simulink model "simultaneous_amp_freq_modulation_simulink"  (R2019a)
settings: Solver=VariableStepAuto  StartTime=0.0  StopTime=10.0  RelTol=1e-3
values from neighbouring files (symbols this model uses):
  fs = 1/Ts    (= 2560)    [Simultaneous_Amp_and_Freq_Modulation_2.m]    (also in Time_Frequency_Power_domain_analysis.m = 850; extended_spectral_analysis.m)
  m = 0.25    [Simultaneous_Amp_and_Freq_Modulation_2.m]    (also in Time_Frequency_Power_domain_analysis.m = 0.5; extended_spectral_analysis.m)
libraries: dspxfrm3 x2, dspsrcs4 x1
settings Model: Creator=HP  LastModifiedBy=PRASHANT
settings DataIOCC: ReturnWorkspaceOutputs=off
settings DebuggingCC: PregeneratedLibrarySubsystemCodeDiagnostic=none  ArithmeticOperatorsInVariantConditions=warning
settings SFSimCC: SimUseLocalCustomCode=off
settings RTWCC: RTWUseLocalCustomCode=off

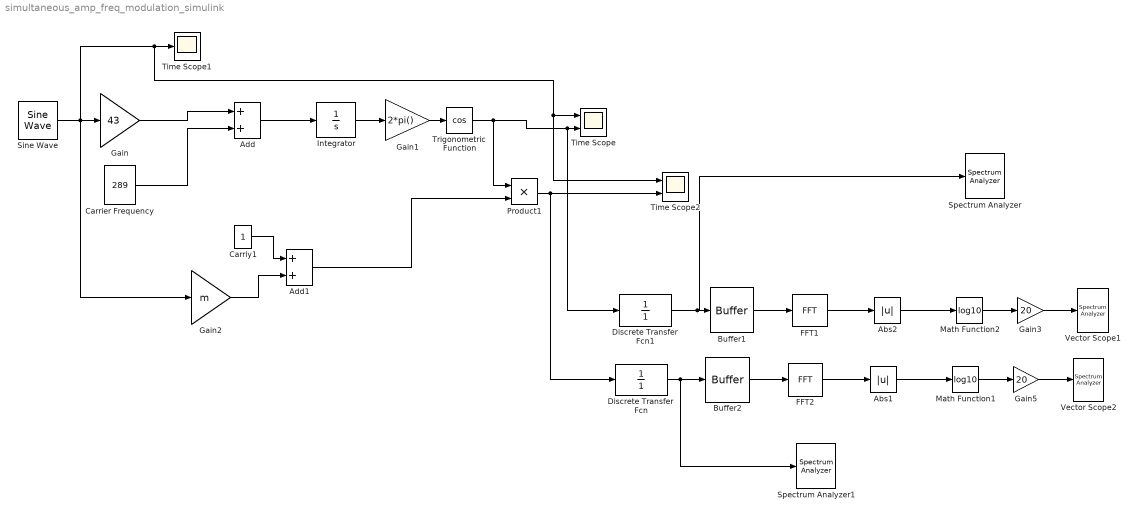
== system simultaneous_amp_freq_modulation_simulink ==
  Abs1 : Abs
  Abs2 : Abs
  Add : Sum
  Add1 : Sum
  Buffer1 : Buffer  N=4096*4
  Buffer2 : Buffer  N=4096*4
  Carrier Frequency : Constant  Value=289
  Carriy1 : Constant
  Discrete Transfer Fcn : DiscreteTransferFcn  Denominator=[1]  SampleTime=1/fs
  Discrete Transfer Fcn1 : DiscreteTransferFcn  Denominator=[1]  SampleTime=1/fs
  FFT1 : dspxfrm3/FFT  FFTImplementation=Auto  CompMethod=Table lookup  TableOpt=NEW  TableOptActive=Speed  BitRevOrder=off  Normalize=on  InheritFFTLength=off  FFTLength=4096  WrapInput=on  roundingMode=Floor  overflowMode=off  firstCoeffDataTypeStr=Inherit: Same word length as input  firstCoeffLastDataTypeStr=Inherit: Same word length as input  outputMin=[]  outputMax=[]
  FFT2 : dspxfrm3/FFT  FFTImplementation=Auto  CompMethod=Table lookup  TableOpt=NEW  TableOptActive=Speed  BitRevOrder=off  Normalize=on  InheritFFTLength=off  FFTLength=4096  WrapInput=on  roundingMode=Floor  overflowMode=off  firstCoeffDataTypeStr=Inherit: Same word length as input  firstCoeffLastDataTypeStr=Inherit: Same word length as input  outputMin=[]  outputMax=[]
  Gain : Gain  Gain=43
  Gain1 : Gain  Gain=2*pi()
  Gain2 : Gain  Gain=m
  Gain3 : Gain  Gain=20
  Gain5 : Gain  Gain=20
  Integrator : Integrator
  Math Function1 : Math  Operator=log10  SaturateOnIntegerOverflow=on
  Math Function2 : Math  Operator=log10  SaturateOnIntegerOverflow=on
  Product1 : Product
  Sine Wave : dspsrcs4/Sine Wave  Amplitude=2  Frequency=50  Phase=0  SampleMode=Discrete  OutComplex=Real  CompMethod=Trigonometric fcn  TableSize=Speed  SampleTime=1/fs  SamplesPerFrame=1  ResetState=Restart at time zero  OutputFrames=off  dataType=double  wordLen=16  udDataType=sfix(16)  fracBitsMode=Best precision  numFracBits=15  OutDataTypeStr=double  LastOutDataTypeStr=double
  Spectrum Analyzer : SpectrumAnalyzer
  Spectrum Analyzer1 : SpectrumAnalyzer
  Time Scope : Scope  NumInputPorts=2
  Time Scope1 : Scope
  Time Scope2 : Scope  NumInputPorts=2
  Trigonometric Function : Trigonometry  Operator=cos
  Vector Scope1 : SpectrumAnalyzer
  Vector Scope2 : SpectrumAnalyzer
  wires:
  Gain/1 -> Add/1
  Carrier Frequency/1 -> Add/2
  Add/1 -> Integrator/1
  Integrator/1 -> Gain1/1
  Gain1/1 -> Trigonometric Function/1
  Carriy1/1 -> Add1/1
  Gain2/1 -> Add1/2
  Add1/1 -> Product1/2
  Sine Wave/1 -> Gain2/1, Time Scope/1, Time Scope2/1, Time Scope1/1, Gain/1
  Product1/1 -> Discrete Transfer Fcn/1, Time Scope2/2
  Buffer2/1 -> FFT2/1
  FFT2/1 -> Abs1/1
  Abs1/1 -> Math Function1/1
  Math Function1/1 -> Gain5/1
  Trigonometric Function/1 -> Product1/1, Discrete Transfer Fcn1/1, Time Scope/2
  Buffer1/1 -> FFT1/1
  Math Function2/1 -> Gain3/1
  FFT1/1 -> Abs2/1
  Abs2/1 -> Math Function2/1
  Gain5/1 -> Vector Scope2/1
  Gain3/1 -> Vector Scope1/1
  Discrete Transfer Fcn1/1 -> Spectrum Analyzer/1, Buffer1/1
  Discrete Transfer Fcn/1 -> Spectrum Analyzer1/1, Buffer2/1
